simulink model "irep_force_control_simu_v2"  (R2015a)
settings: Solver=ode3  StartTime=0.0  StopTime=inf  FixedStep=dt  RelTol=1e-3
InitFcn:
  | IREP_DEPENDENCY
  | init_omni
  | init_filters
  | init_invivo
  | init_telemanipulation
  | init_parker_xyz
  | init_magnetic_tracker
  | init_loadcell
  | init_scopes
  | init_homing
  | init_force_control
  | init_xpc_invivo_simu
undefined symbols (not defined in the file or in its folder): ang_vel_scale, B_simu, beta, camera_home_voltage, counter_offset, dt, dt_trakstar, E_Y, encoder_counts, epsilon_robust_inverse, FS_LUT, gear_ratio, HomingFineEps, HomingRoughEps, HomingRoughVelocity, I1_primary, I1_secondary, I2_primary, I2_secondary, irep_parameters_left, irep_parameters_right, joystick_filter_coeffs, K_d, K_i, K_naive_inv, K_p, k_right, L1l, L1r, L2l, L2r, L_zeus, left_arm_home_voltage, left_x0_parallelogram, LeftArmHomingDirectionVector, LeftArmHomingIntGain, lin_vel_scale, LOADCELL_BIAS, LOADCELL_GAIN, max_conf_space_speed, N_joystick, N_pots, N_trakstar, OmegaMax, OmegaMin, orientation_epsilon, position_epsilon, pots_filter_coeffs, q_eps_backlash, quadrature_mode, r, right_arm_home_voltage, RightArmHomingDirectionVector, RightArmHomingIntGain, screw_pitch, statics_param, tau_compression_bias, tau_compression_gains, tau_neutral_deadband, tau_tension_bias ... (+15)
libraries: slrtlib x39, xpcrtudplib x13, xpcobsoletelib x13, simulink x8, dspswit3 x2, dspsigops x1
(part 3 of 6)

== system irep_force_control_simu_v2/In-Vivo System/motor simulation/q_des to q_cur mapping ==
  q cur in : Inport
  Bus Creator1 : BusCreator  Inputs=23
  Bus Selector : BusSelector  OutputSignals=Right arm - Proximal Segment Y,Right arm - Gripper Joint,Right arm - Proximal Segment X,Right arm - Distal Segment X,Right arm - Wrist Joint,Right arm - Distal Segment Y,Right arm - Parallelogram Deploy,Right arm - Parallelogram Insert,Left arm - Proximal Segment Y,Left arm - Gripper Joint,Left arm - Proximal Segment X,Left arm - Distal Segment X,Left arm - Wrist Joint,Left arm - Distal Segment Y,Left arm - Parallelogram Deploy,Left arm - Parallelogram Insert,Righ arm - Overall Translational Movement,Left arm - Overall Translational Movement,Camera shell open,Camera Pan,Camera Tilt,Parker insertion stage,Parker rotary stage
  Demux : Demux  Outputs=23
  Mux : Mux  Inputs=23
  q cur out : Outport
  wires:
  Demux/1 -> Bus Creator1/1  "Righ arm - Overall Translational Movement"
  Demux/2 -> Bus Creator1/2  "Right arm - Parallelogram Insert"
  Demux/3 -> Bus Creator1/3  "Right arm - Parallelogram Deploy"
  Demux/4 -> Bus Creator1/4  "Right arm - Proximal Segment X"
  Demux/5 -> Bus Creator1/5  "Right arm - Proximal Segment Y"
  Demux/6 -> Bus Creator1/6  "Right arm - Distal Segment X"
  Demux/7 -> Bus Creator1/7  "Right arm - Distal Segment Y"
  Demux/8 -> Bus Creator1/8  "Right arm - Wrist Joint"
  Demux/9 -> Bus Creator1/9  "Right arm - Gripper Joint"
  Demux/10 -> Bus Creator1/10  "Left arm - Overall Translational Movement"
  Demux/11 -> Bus Creator1/11  "Left arm - Parallelogram Insert"
  Demux/12 -> Bus Creator1/12  "Left arm - Parallelogram Deploy"
  Demux/13 -> Bus Creator1/13  "Left arm - Proximal Segment X"
  Demux/14 -> Bus Creator1/14  "Left arm - Proximal Segment Y"
  Demux/15 -> Bus Creator1/15  "Left arm - Distal Segment X"
  Demux/16 -> Bus Creator1/16  "Left arm - Distal Segment Y"
  Demux/17 -> Bus Creator1/17  "Left arm - Wrist Joint"
  Demux/18 -> Bus Creator1/18  "Left arm - Gripper Joint"
  Demux/19 -> Bus Creator1/19  "Camera shell open"
  Demux/20 -> Bus Creator1/20  "Camera Pan"
  Demux/21 -> Bus Creator1/21  "Camera Tilt"
  Demux/22 -> Bus Creator1/22  "Parker insertion stage"
  Demux/23 -> Bus Creator1/23  "Parker rotary stage"
  Bus Creator1/1 -> Bus Selector/1
  Bus Selector/1 -> Mux/1  "<Right arm - Proximal Segment Y>"
  Bus Selector/2 -> Mux/2  "<Right arm - Gripper Joint>"
  Bus Selector/3 -> Mux/3  "<Right arm - Proximal Segment X>"
  Bus Selector/4 -> Mux/4  "<Right arm - Distal Segment X>"
  Bus Selector/5 -> Mux/5  "<Right arm - Wrist Joint>"
  Bus Selector/6 -> Mux/6  "<Right arm - Distal Segment Y>"
  Bus Selector/7 -> Mux/7  "<Right arm - Parallelogram Deploy>"
  Bus Selector/8 -> Mux/8  "<Right arm - Parallelogram Insert>"
  Bus Selector/9 -> Mux/9  "<Left arm - Proximal Segment Y>"
  Bus Selector/10 -> Mux/10  "<Left arm - Gripper Joint>"
  Bus Selector/11 -> Mux/11  "<Left arm - Proximal Segment X>"
  Bus Selector/12 -> Mux/12  "<Left arm - Distal Segment X>"
  Bus Selector/13 -> Mux/13  "<Left arm - Wrist Joint>"
  Bus Selector/14 -> Mux/14  "<Left arm - Distal Segment Y>"
  Bus Selector/15 -> Mux/15  "<Left arm - Parallelogram Deploy>"
  Bus Selector/16 -> Mux/16  "<Left arm - Parallelogram Insert>"
  Bus Selector/17 -> Mux/17  "<Righ arm - Overall Translational Movement>"
  Bus Selector/18 -> Mux/18  "<Left arm - Overall Translational Movement>"
  Bus Selector/19 -> Mux/19  "<Camera shell open>"
  Bus Selector/20 -> Mux/20  "<Camera Pan>"
  Bus Selector/21 -> Mux/21  "<Camera Tilt>"
  Bus Selector/22 -> Mux/22  "<Parker insertion stage>"
  Bus Selector/23 -> Mux/23  "<Parker rotary stage>"
  q cur in/1 -> Demux/1
  Mux/1 -> q cur out/1

== system irep_force_control_simu_v2/In-Vivo System/motor simulation/u mapping ==
  u in : Inport
  Bus Selector : BusSelector  OutputSignals=Righ arm - Overall Translational Movement,Right arm - Parallelogram Insert,Right arm - Parallelogram Deploy,Right arm - Proximal Segment X,Right arm - Proximal Segment Y,Right arm - Distal Segment X,Right arm - Distal Segment Y,Right arm - Wrist Joint,Right arm - Gripper Joint,Left arm - Overall Translational Movement,Left arm - Parallelogram Insert,Left arm - Parallelogram Deploy,Left arm - Proximal Segment X,Left arm - Proximal Segment Y,Left arm - Distal Segment X,Left arm - Distal Segment Y,Left arm - Wrist Joint,Left arm - Gripper Joint,Camera shell open,Camera Pan,Camera Tilt,Parker insertion stage,Parker rotary stage
  Mux : Mux  Inputs=23
  u out : Outport
  wires:
  Bus Selector/1 -> Mux/1  "<Righ arm - Overall Translational Movement>"
  Bus Selector/2 -> Mux/2  "<Right arm - Parallelogram Insert>"
  Bus Selector/3 -> Mux/3  "<Right arm - Parallelogram Deploy>"
  Bus Selector/4 -> Mux/4  "<Right arm - Proximal Segment X>"
  Bus Selector/5 -> Mux/5  "<Right arm - Proximal Segment Y>"
  Bus Selector/6 -> Mux/6  "<Right arm - Distal Segment X>"
  Bus Selector/7 -> Mux/7  "<Right arm - Distal Segment Y>"
  Bus Selector/8 -> Mux/8  "<Right arm - Wrist Joint>"
  Bus Selector/9 -> Mux/9  "<Right arm - Gripper Joint>"
  Bus Selector/10 -> Mux/10  "<Left arm - Overall Translational Movement>"
  Bus Selector/11 -> Mux/11  "<Left arm - Parallelogram Insert>"
  Bus Selector/12 -> Mux/12  "<Left arm - Parallelogram Deploy>"
  Bus Selector/13 -> Mux/13  "<Left arm - Proximal Segment X>"
  Bus Selector/14 -> Mux/14  "<Left arm - Proximal Segment Y>"
  Bus Selector/15 -> Mux/15  "<Left arm - Distal Segment X>"
  Bus Selector/16 -> Mux/16  "<Left arm - Distal Segment Y>"
  Bus Selector/17 -> Mux/17  "<Left arm - Wrist Joint>"
  Bus Selector/18 -> Mux/18  "<Left arm - Gripper Joint>"
  Bus Selector/19 -> Mux/19  "<Camera shell open>"
  Bus Selector/20 -> Mux/20  "<Camera Pan>"
  Bus Selector/21 -> Mux/21  "<Camera Tilt>"
  Bus Selector/22 -> Mux/22  "<Parker insertion stage>"
  Bus Selector/23 -> Mux/23  "<Parker rotary stage>"
  u in/1 -> Bus Selector/1
  Mux/1 -> u out/1

== system irep_force_control_simu_v2/Joint Level PID Control in mm/Bus selector/Camera selector ==
  In1 : Inport
  Bus Selector : BusSelector  OutputSignals=q.Camera shell open,q.Camera Pan,q.Camera Tilt
  Mux : Mux  Inputs=3
  Out1 : Outport
  wires:
  Mux/1 -> Out1/1
  In1/1 -> Bus Selector/1
  Bus Selector/3 -> Mux/3  "<Camera Tilt>"
  Bus Selector/2 -> Mux/2  "<Camera Pan>"
  Bus Selector/1 -> Mux/1  "<Camera shell open>"

== system irep_force_control_simu_v2/Joint Level PID Control in mm/Bus selector/Left arm selector ==
  In1 : Inport
  Bus Selector : BusSelector  OutputSignals=q.Left arm - overall translational movement,q.Left arm - parallelogram insert joint,q.Left arm - parallelogram deployment joint,q.Left arm - proximal segment - bending in X,q.Left arm - proximal segment - bending in Y,q.Left arm - distal segment - bending in x,q.Left arm - distal segment - bending in y,q.Left arm - wrist,q.Left arm - gripper joint
  Mux : Mux  Inputs=9
  Out1 : Outport
  wires:
  In1/1 -> Bus Selector/1
  Mux/1 -> Out1/1
  Bus Selector/1 -> Mux/1  "<Left arm - overall translational movement>"
  Bus Selector/2 -> Mux/2  "<Left arm - parallelogram insert joint>"
  Bus Selector/3 -> Mux/3  "<Left arm - parallelogram deployment joint>"
  Bus Selector/4 -> Mux/4  "<Left arm - proximal segment - bending in X>"
  Bus Selector/5 -> Mux/5  "<Left arm - proximal segment - bending in Y>"
  Bus Selector/8 -> Mux/8  "<Left arm - wrist>"
  Bus Selector/9 -> Mux/9  "<Left arm - gripper joint>"
  Bus Selector/6 -> Mux/6  "<Left arm - distal segment - bending in x>"
  Bus Selector/7 -> Mux/7  "<Left arm - distal segment - bending in y>"

== system irep_force_control_simu_v2/Joint Level PID Control in mm/Bus selector/RZ ==
  In1 : Inport
  Bus Selector : BusSelector  OutputSignals=q.Parker insertion stage,q.Parker rotary stage
  Mux : Mux  Inputs=2
  Out1 : Outport
  wires:
  Mux/1 -> Out1/1
  In1/1 -> Bus Selector/1
  Bus Selector/2 -> Mux/2  "<Parker rotary stage>"
  Bus Selector/1 -> Mux/1  "<Parker insertion stage>"

== system irep_force_control_simu_v2/Joint Level PID Control in mm/Bus selector/Right arm selector ==
  In1 : Inport
  Bus Selector : BusSelector  OutputSignals=q.Right arm - overall translational movement,q.Right arm - parallelogram insert joint,q.Right arm - parallelogram deployment joint,q.Right arm - Proximal segment - bending in X,q.Righ arm - Proximal segment - bending in Y,q.Right arm - distal segment - bending in X,q.Right arm - distal segment - bending in Y,q.Right arm - wrist,q.Right arm - Gripper Joint
  Mux : Mux  Inputs=9
  Out1 : Outport
  wires:
  In1/1 -> Bus Selector/1
  Mux/1 -> Out1/1
  Bus Selector/1 -> Mux/1  "<Right arm - overall translational movement>"
  Bus Selector/2 -> Mux/2  "<Right arm - parallelogram insert joint>"
  Bus Selector/3 -> Mux/3  "<Right arm - parallelogram deployment joint>"
  Bus Selector/4 -> Mux/4  "<Right arm - Proximal segment - bending in X>"
  Bus Selector/5 -> Mux/5  "<Righ arm - Proximal segment - bending in Y>"
  Bus Selector/6 -> Mux/6  "<Right arm - distal segment - bending in X>"
  Bus Selector/7 -> Mux/7  "<Right arm - distal segment - bending in Y>"
  Bus Selector/8 -> Mux/8  "<Right arm - wrist>"
  Bus Selector/9 -> Mux/9  "<Right arm - Gripper Joint>"

== system irep_force_control_simu_v2/Scopes/Friction Estimation Data UDP/Right arm joint def ==
  sensors : Inport
  Bus Selector4 : BusSelector  OutputSignals=q.Right arm - overall translational movement,q.Right arm - parallelogram insert joint,q.Right arm - parallelogram deployment joint,q.Right arm - Proximal segment - bending in X,q.Righ arm - Proximal segment - bending in Y,q.Right arm - distal segment - bending in X,q.Right arm - distal segment - bending in Y,q.Right arm - wrist,q.Right arm - Gripper Joint
  Mux1 : Mux  Inputs=9
  right q_cur : Outport
  wires:
  Bus Selector4/1 -> Mux1/1  "<Right arm - overall translational movement>"
  Bus Selector4/2 -> Mux1/2  "<Right arm - parallelogram insert joint>"
  Bus Selector4/3 -> Mux1/3  "<Right arm - parallelogram deployment joint>"
  Bus Selector4/4 -> Mux1/4  "<Right arm - Proximal segment - bending in X>"
  Bus Selector4/5 -> Mux1/5  "<Righ arm - Proximal segment - bending in Y>"
  Bus Selector4/6 -> Mux1/6  "<Right arm - distal segment - bending in X>"
  Bus Selector4/7 -> Mux1/7  "<Right arm - distal segment - bending in Y>"
  Bus Selector4/8 -> Mux1/8  "<Right arm - wrist>"
  Bus Selector4/9 -> Mux1/9  "<Right arm - Gripper Joint>"
  sensors/1 -> Bus Selector4/1
  Mux1/1 -> right q_cur/1

== system irep_force_control_simu_v2/Trajectory Planner/Camera/Homing Procedure ==
  sensors : Inport
  Enable : EnablePort
  Bus Selector : BusSelector  OutputSignals=A/D signals.camera pots
  Discrete-Time Integrator : DiscreteIntegrator  InitialCondition=zeros(3,1)  SampleTime=dt
  Gain : Gain  Gain=[0.1 0.1 0.1]  SampleTime=dt
  Homing Completion : MATLAB Function  TreatAsAtomicUnit=on
  Sum : Sum  Inputs=|+-  SampleTime=dt
  Terminator1 : Terminator
  home voltage : Constant  Value=camera_home_voltage  SampleTime=dt
  q des : Outport
  wires:
  sensors/1 -> Bus Selector/1
  home voltage/1 -> Sum/1
  Bus Selector/1 -> Sum/2  "<camera pots>"
  Sum/1 -> Gain/1, Homing Completion/1(u)
  Gain/1 -> Discrete-Time Integrator/1
  Discrete-Time Integrator/1 -> q des/1
  Homing Completion/1(y) -> Terminator1/1

== system irep_force_control_simu_v2/Trajectory Planner/Camera/Joint Space ==
  Enable : EnablePort
  q des : Constant  Value=zeros(3,1)  SampleTime=dt
  Out1 : Outport
  wires:
  q des/1 -> Out1/1

== system irep_force_control_simu_v2/Trajectory Planner/Camera/Joystick Control for Cam ==
  sensors : Inport
  Enable : EnablePort
  Bus Selector : BusSelector  OutputSignals=A/D signals.camera joystick
  Demux : Demux  Outputs=3
  Discrete-Time Integrator : DiscreteIntegrator  SampleTime=dt  LimitOutput=on  UpperSaturationLimit=[3;3;3]  LowerSaturationLimit=[-3;-3;-3]
  Gain : Gain  Gain=diag([0.3 0.3 0.3])  Multiplication=Matrix(K*u)  SampleTime=dt
  Gain1 : Gain  Gain=-1
  Mux : Mux  Inputs=3
  q des : Outport
  wires:
  sensors/1 -> Bus Selector/1
  Gain/1 -> Discrete-Time Integrator/1
  Discrete-Time Integrator/1 -> q des/1
  Bus Selector/1 -> Demux/1  "<camera joystick>"
  Mux/1 -> Gain/1
  Demux/2 -> Gain1/1
  Demux/1 -> Mux/2
  Demux/3 -> Mux/1
  Gain1/1 -> Mux/3

== system irep_force_control_simu_v2/Trajectory Planner/Camera/Tool Tracking ==
  tool XY : Inport
  Enable : EnablePort
  Constant1 : Constant  Value=0  SampleTime=dt
  Discrete-Time Integrator : DiscreteIntegrator  SampleTime=dt  LimitOutput=on  UpperSaturationLimit=[3;3]  LowerSaturationLimit=[-3;-3]
  Gain : Gain  Gain=[0.01,0.01]  SampleTime=dt
  Mux : Mux  Inputs=2
  q des : Outport
  wires:
  tool XY/1 -> Gain/1
  Mux/1 -> q des/1
  Constant1/1 -> Mux/1
  Gain/1 -> Discrete-Time Integrator/1
  Discrete-Time Integrator/1 -> Mux/2

== system irep_force_control_simu_v2/Trajectory Planner/Left Arm/High Level ==
  Master : Inport
  sensors : Inport  Port=2
  Enable : EnablePort
  Actuation Compensation : Subsystem  TreatAsAtomicUnit=on
  Add : Sum
  Configuration Space : Subsystem  TreatAsAtomicUnit=on
  Enable Compensation : Constant  Value=0  SampleTime=dt
  Enable Configuration Space : Constant  Value=0  SampleTime=dt
  Enable Task Space : Constant  Value=0  SampleTime=dt
  Inverse Istantaneous Kinematics : Subsystem
  Merge : Merge  InitialOutput=zeros(8,1)
  Task Space : Subsystem  TreatAsAtomicUnit=on
  q des : Outport
  conf space : Outport  Port=2
  b0_dot_left : Outport  Port=3
  TASK_EN : Outport  Port=4
  current_pose : Outport  Port=5
  wires:
  Enable Task Space/1 -> TASK_EN/1, Task Space/Enable
  Task Space/1("b1 dot, psi dot") -> Merge/2
  Master/1 -> Task Space/1(Master), Inverse Istantaneous Kinematics/3(Master)
  Inverse Istantaneous Kinematics/2(conf space) -> Actuation Compensation/2(conf space), Task Space/2("b1 curr, psi curr"), conf space/1
  Inverse Istantaneous Kinematics/1(q des) -> Actuation Compensation/1(q des), Add/1
  Add/1 -> q des/1
  Actuation Compensation/1(epsilon) -> Add/2
  Enable Compensation/1 -> Actuation Compensation/Enable
  Enable Configuration Space/1 -> Configuration Space/Enable
  Configuration Space/1("b1 dot, psi dot") -> Merge/1
  sensors/1 -> Inverse Istantaneous Kinematics/2(sensors), Task Space/3(sensors)
  Merge/1 -> Inverse Istantaneous Kinematics/1(In1)
  Inverse Istantaneous Kinematics/3(b0 dot left) -> b0_dot_left/1
  Task Space/2(current_pose) -> current_pose/1

== system irep_force_control_simu_v2/Trajectory Planner/Left Arm/Low Level ==
  sensors : Inport
  Enable : EnablePort
  Bus Selector : BusSelector  OutputSignals=Pots_Connect.L_Pots_Connect
  Enable Home Procedure : Constant  Value=0  SampleTime=dt
  Enable Joint Space : Constant  Value=0  SampleTime=dt
  Home Procedure : Subsystem  TreatAsAtomicUnit=on
  Joint Space : Subsystem  TreatAsAtomicUnit=on
  Merge1 : Merge  InitialOutput=zeros(9,1)
  Not And : MATLAB Function  TreatAsAtomicUnit=on
  q des : Outport
  wires:
  sensors/1 -> Bus Selector/1, Home Procedure/1(sensors)
  Merge1/1 -> q des/1
  Enable Joint Space/1 -> Joint Space/Enable
  Joint Space/1(q des) -> Merge1/2
  Bus Selector/1 -> Not And/1(connected)  "<L_Pots_Connect>"
  Enable Home Procedure/1 -> Not And/2(enable_home)
  Not And/1(enable) -> Home Procedure/Enable
  Home Procedure/1(q des) -> Merge1/1

== system irep_force_control_simu_v2/Trajectory Planner/RZ/Joystick Control for RZ ==
  sensors : Inport
  Enable : EnablePort
  Bus Selector : BusSelector  OutputSignals=A/D signals.camera joystick
  Embedded MATLAB Function : MATLAB Function  TreatAsAtomicUnit=on
  Gain : Gain  Gain=diag(-[2 0 0.005])  Multiplication=Matrix(K*u)  SampleTime=dt
  q des : Outport
  wires:
  sensors/1 -> Bus Selector/1
  Gain/1 -> q des/1
  Embedded MATLAB Function/1(y) -> Gain/1
  Bus Selector/1 -> Embedded MATLAB Function/1(u)  "<camera joystick>"

== system irep_force_control_simu_v2/Trajectory Planner/RZ/Subsystem ==
  In1 : Inport
  Demux : Demux  Outputs=3
  Mux : Mux  Inputs=2
  Terminator : Terminator
  Out1 : Outport
  wires:
  Demux/1 -> Mux/1
  Demux/3 -> Mux/2
  Demux/2 -> Terminator/1
  In1/1 -> Demux/1
  Mux/1 -> Out1/1

== system irep_force_control_simu_v2/Trajectory Planner/Right Arm/High Level ==
  Master : Inport
  sensors : Inport  Port=2
  Enable : EnablePort
  Actuation Compensation : Subsystem  TreatAsAtomicUnit=on
  Add : Sum
  Configuration Space : Subsystem  TreatAsAtomicUnit=on
  Enable Compensation : Constant  Value=0  SampleTime=dt
  Enable Configuration Space : Constant  Value=0  SampleTime=dt
  Enable Task Space : Constant  Value=0  SampleTime=dt
  Inverse Istantaneous Kinematics : Subsystem
  Merge : Merge  InitialOutput=zeros(8,1)
  Right eps : slrtlib/Displays and Logging/Scope   scopeno=32  scopetype=Host  autostart=on  viewmode=Numerical  formatstr=scope_format_right_q_des  grid=on  ylimits=[0,0]  nosamples=10  noprepostsamples=0  interleave=1  triggermode=FreeRun  triggersignal=1  trigsignalfromport=off  triggerlevel=0.0  triggerslope=Either  triggerscope=1  triggersample=0  filename=weights.dat  mode=Lazy  writesize=512  autorestart=off  dynamicfilemode=off  maxwritefilesize=512*1024^2
  Task Space : Subsystem  TreatAsAtomicUnit=on
  delay : Subsystem
  q des : Outport
  conf space : Outport  Port=2  PortDimensions=8
  b0 dot : Outport  Port=3  PortDimensions=1
  TASK_EN : Outport  Port=4
  current_pose : Outport  Port=5
  q dot sgn : Outport  Port=6
  wires:
  Merge/1 -> [psi_dot], Inverse Istantaneous Kinematics/1(PSI dot)
  Enable Task Space/1 -> TASK_EN/1, Task Space/Enable
  Task Space/1("b0 dot, b1 dot, psi dot") -> Merge/2
  Master/1 -> Task Space/1(Master), Inverse Istantaneous Kinematics/3(Master)
  Inverse Istantaneous Kinematics/2(conf space) -> Actuation Compensation/2(conf space), Task Space/2("b1 curr, psi curr"), conf space/1
  Configuration Space/1("b1 dot, psi dot") -> Merge/1
  Inverse Istantaneous Kinematics/1(q des) -> Add/1, delay/1(In1)
  Actuation Compensation/1(epsilon) -> Add/2, Right eps/1
  Enable Compensation/1 -> Actuation Compensation/Enable
  sensors/1 -> Task Space/3(sensors), Inverse Istantaneous Kinematics/2(sensors)
  Inverse Istantaneous Kinematics/3(b0_dot_right) -> b0 dot/1
  Add/1 -> q des/1
  Task Space/2(current_pose) -> current_pose/1
  Enable Configuration Space/1 -> Configuration Space/Enable
  [psi_dot] -> Actuation Compensation/3(psi dot)
  delay/1(Out1) -> Actuation Compensation/1(q des)
  Actuation Compensation/2(q dot sgn) -> q dot sgn/1

== system irep_force_control_simu_v2/Trajectory Planner/Right Arm/Low Level ==
  sensors : Inport
  Enable : EnablePort
  Bus Selector : BusSelector  OutputSignals=Pots_Connect.R_Pots_Connect
  Enable Home Procedure : Constant  Value=0  SampleTime=dt
  Enable Joint Space : Constant  Value=0  SampleTime=dt
  Home Procedure : Subsystem  TreatAsAtomicUnit=on
  Joint Space : Subsystem  TreatAsAtomicUnit=on
  Merge1 : Merge  InitialOutput=zeros(9,1)
  Not And : MATLAB Function  TreatAsAtomicUnit=on
  q des : Outport
  wires:
  sensors/1 -> Home Procedure/1(sensors), Bus Selector/1
  Home Procedure/1(q des) -> Merge1/1
  Enable Joint Space/1 -> Joint Space/Enable
  Joint Space/1(q des) -> Merge1/2
  Merge1/1 -> q des/1
  Bus Selector/1 -> Not And/1(connected)  "<R_Pots_Connect>"
  Not And/1(enable) -> Home Procedure/Enable
  Enable Home Procedure/1 -> Not And/2(enable_home)

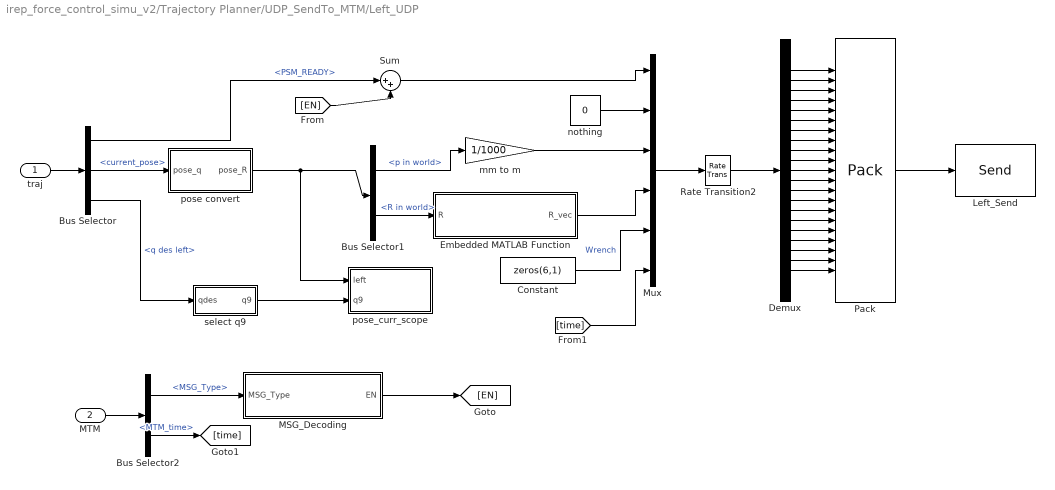
== system irep_force_control_simu_v2/Trajectory Planner/UDP_SendTo_MTM/Left_UDP ==
  traj : Inport
  MTM : Inport  Port=2
  Bus Selector : BusSelector  OutputSignals=left arm.PSM_READY,left arm.current_pose,left arm.q des left
  Bus Selector1 : BusSelector  OutputSignals=p in world,R in world
  Bus Selector2 : BusSelector  OutputSignals=MSG_Type,MTM_time
  Constant : Constant  Value=zeros(6,1)
  Demux : Demux  Outputs=21
  Embedded MATLAB Function : MATLAB Function  TreatAsAtomicUnit=on
  Left_Send : xpcrtudplib/Legacy UDP/Send   ipAddress=192.168.1.104  ipPort=10004  localPort=-1  vblLen=off  sampletime=dt_omni
  MSG_Decoding : MATLAB Function  TreatAsAtomicUnit=on
  Mux : Mux  Inputs=6
  Pack : xpcobsoletelib/Utilities/Pack   datatypes={'double' 'double' 'double' 'double' 'double' 'double' 'double' 'double' 'double' 'double' 'double' 'double' 'double' 'double' 'double' 'double' 'double' 'double' 'double' 'double' 'double'}  byteAlign=1
  Rate Transition2 : RateTransition  OutPortSampleTime=dt_omni
  Sum : Sum  Inputs=|++
  mm to m : Gain  Gain=1/1000
  nothing : Constant  Value=0
  pose convert : Subsystem
  pose_curr_scope : Subsystem
  select q9 : Subsystem
  wires:
  pose convert/1(pose_R) -> Bus Selector1/1, pose_curr_scope/1(left)
  Bus Selector/2 -> pose convert/1(pose_q)  "<current_pose>"
  Constant/1 -> Mux/5  "Wrench"
  Demux/21 -> Pack/21
  Demux/20 -> Pack/20
  Demux/19 -> Pack/19
  Demux/18 -> Pack/18
  Demux/17 -> Pack/17
  Demux/16 -> Pack/16
  Demux/15 -> Pack/15
  Demux/14 -> Pack/14
  Demux/13 -> Pack/13
  Demux/12 -> Pack/12
  Demux/11 -> Pack/11
  Demux/10 -> Pack/10
  Demux/9 -> Pack/9
  Demux/8 -> Pack/8
  Demux/7 -> Pack/7
  Demux/6 -> Pack/6
  Demux/5 -> Pack/5
  Demux/4 -> Pack/4
  Demux/3 -> Pack/3
  Demux/2 -> Pack/2
  Demux/1 -> Pack/1
  [time] -> Mux/6
  Sum/1 -> Mux/1
  [EN] -> Sum/2
  Bus Selector/1 -> Sum/1  "<PSM_READY>"
  nothing/1 -> Mux/2
  MSG_Decoding/1(EN) -> [EN]
  Bus Selector2/2 -> [time]  "<MTM_time>"
  Bus Selector2/1 -> MSG_Decoding/1(MSG_Type)  "<MSG_Type>"
  MTM/1 -> Bus Selector2/1
  select q9/1(q9) -> pose_curr_scope/2(q9)
  Bus Selector/3 -> select q9/1(qdes)  "<q des left>"
  mm to m/1 -> Mux/3
  traj/1 -> Bus Selector/1
  Embedded MATLAB Function/1(R_vec) -> Mux/4
  Bus Selector1/1 -> mm to m/1  "<p in world>"
  Rate Transition2/1 -> Demux/1
  Mux/1 -> Rate Transition2/1
  Pack/1 -> Left_Send/1
  Bus Selector1/2 -> Embedded MATLAB Function/1(R)  "<R in world>"

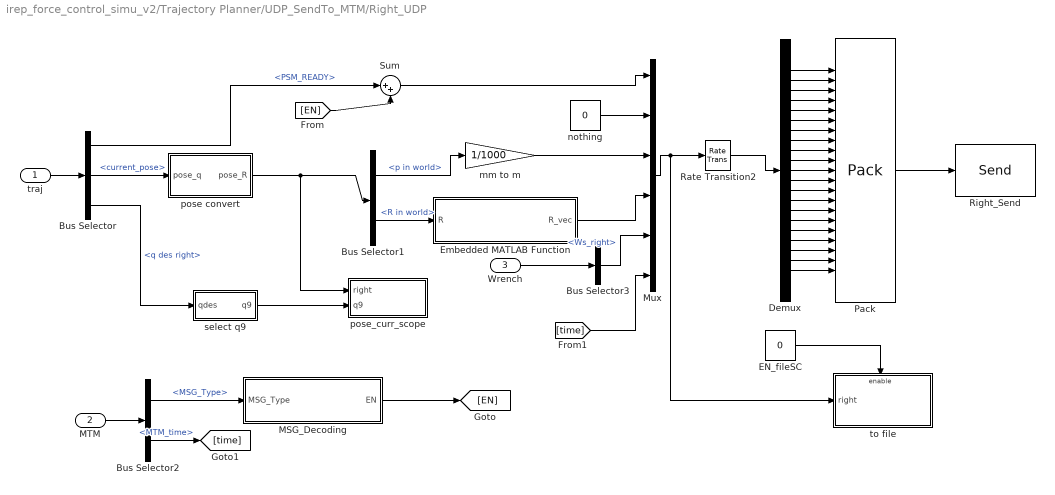
== system irep_force_control_simu_v2/Trajectory Planner/UDP_SendTo_MTM/Right_UDP ==
  traj : Inport
  MTM : Inport  Port=2
  Wrench : Inport  Port=3
  Bus Selector : BusSelector  OutputSignals=right arm.PSM_READY,right arm.current_pose,right arm.q des right
  Bus Selector1 : BusSelector  OutputSignals=p in world,R in world
  Bus Selector2 : BusSelector  OutputSignals=MSG_Type,MTM_time
  Bus Selector3 : BusSelector  OutputSignals=Ws_right
  Demux : Demux  Outputs=21
  EN_fileSC : Constant  Value=0
  Embedded MATLAB Function : MATLAB Function  TreatAsAtomicUnit=on
  MSG_Decoding : MATLAB Function  TreatAsAtomicUnit=on
  Mux : Mux  Inputs=6
  Pack : xpcobsoletelib/Utilities/Pack   datatypes={'double' 'double' 'double' 'double' 'double' 'double' 'double' 'double' 'double' 'double' 'double' 'double' 'double' 'double' 'double' 'double' 'double' 'double' 'double' 'double' 'double'}  byteAlign=1
  Rate Transition2 : RateTransition  OutPortSampleTime=dt_omni
  Right_Send : xpcrtudplib/Legacy UDP/Send   ipAddress=192.168.1.104  ipPort=10005  localPort=-1  vblLen=off  sampletime=dt_omni
  Sum : Sum  Inputs=|++
  mm to m : Gain  Gain=1/1000
  nothing : Constant  Value=0
  pose convert : Subsystem
  pose_curr_scope : Subsystem
  select q9 : Subsystem
  to file : Subsystem
  wires:
  Bus Selector1/2 -> Embedded MATLAB Function/1(R)  "<R in world>"
  Pack/1 -> Right_Send/1
  Mux/1 -> Rate Transition2/1, to file/1(right)
  Rate Transition2/1 -> Demux/1
  Bus Selector1/1 -> mm to m/1  "<p in world>"
  Embedded MATLAB Function/1(R_vec) -> Mux/4
  traj/1 -> Bus Selector/1
  mm to m/1 -> Mux/3
  Bus Selector/3 -> select q9/1(qdes)  "<q des right>"
  select q9/1(q9) -> pose_curr_scope/2(q9)
  MTM/1 -> Bus Selector2/1
  Bus Selector2/1 -> MSG_Decoding/1(MSG_Type)  "<MSG_Type>"
  Bus Selector2/2 -> [time]  "<MTM_time>"
  MSG_Decoding/1(EN) -> [EN]
  EN_fileSC/1 -> to file/Enable
  nothing/1 -> Mux/2
  Bus Selector/1 -> Sum/1  "<PSM_READY>"
  [EN] -> Sum/2
  Sum/1 -> Mux/1
  [time] -> Mux/6
  Demux/1 -> Pack/1
  Demux/2 -> Pack/2
  Demux/3 -> Pack/3
  Demux/4 -> Pack/4
  Demux/5 -> Pack/5
  Demux/6 -> Pack/6
  Demux/7 -> Pack/7
  Demux/8 -> Pack/8
  Demux/9 -> Pack/9
  Demux/10 -> Pack/10
  Demux/11 -> Pack/11
  Demux/12 -> Pack/12
  Demux/13 -> Pack/13
  Demux/14 -> Pack/14
  Demux/15 -> Pack/15
  Demux/16 -> Pack/16
  Demux/17 -> Pack/17
  Demux/18 -> Pack/18
  Demux/19 -> Pack/19
  Demux/20 -> Pack/20
  Demux/21 -> Pack/21
  Wrench/1 -> Bus Selector3/1
  Bus Selector3/1 -> Mux/5  "<Ws_right>"
  Bus Selector/2 -> pose convert/1(pose_q)  "<current_pose>"
  pose convert/1(pose_R) -> Bus Selector1/1, pose_curr_scope/1(right)

== system irep_force_control_simu_v2/Wrench Estimation/Wrench Est Right Arm/sel param ==
  note: irep_parameters_right = [Y_OFFSET;L1r;L2r;p_gripper];
  In : Inport
  Demux : Demux  Outputs=[1,1,1,3]
  Mux1 : Mux  Inputs=2
  Terminator : Terminator
  Terminator1 : Terminator
  L : Outport
  wires:
  In/1 -> Demux/1
  Mux1/1 -> L/1
  Demux/2 -> Mux1/1  "L1"
  Demux/3 -> Mux1/2  "L2"
  Demux/1 -> Terminator/1  "Y_OFFSET"
  Demux/4 -> Terminator1/1  "p_gripper"

== system irep_force_control_simu_v2/Wrench Estimation/tau sensing compensation/tau sensing compensation LUT ==
  note: 1st Segment tau bias
  note: 2nd Segment tau bias
  note: Inputs
  tau_measured : Inport
  q_dot_sign : Inport  Port=2
  psi : Inport  Port=3
  Enable : EnablePort
  Constant : Constant  Value=zeros(4,1)
  Demux : Demux  Outputs=[4,4]
  Demux1 : Demux  Outputs=[2,2]
  Mux : Mux  Inputs=2
  Sum : Sum  Inputs=|+-
  Terminator : Terminator
  Terminator1 : Terminator
  tau seg2 bias LUT : Subsystem
  tau_comp : Outport
  wires:
  psi/1 -> Demux1/1
  q_dot_sign/1 -> Demux/1
  Demux1/1 -> [psi1]
  Demux1/2 -> [psi2]
  [psi1] -> Terminator/1
  Demux/1 -> [qdot_sgn1]
  Demux/2 -> [qdot_sgn2]
  [qdot_sgn1] -> Terminator1/1
  tau_measured/1 -> [tau_measured]
  [psi2] -> tau seg2 bias LUT/2(psi seg2)
  [qdot_sgn2] -> tau seg2 bias LUT/1(q dot seg2)
  Constant/1 -> Mux/1
  tau seg2 bias LUT/1(tau bias seg2) -> Mux/2
  Mux/1 -> Sum/2  "tau bias"
  [tau_measured] -> Sum/1
  Sum/1 -> tau_comp/1

== system irep_force_control_simu_v2/Wrench Estimation/tau sensing compensation/tau sensing compensation gain model ==
  q_bb : Inport
  tau_sensed : Inport  Port=2
  Enable : EnablePort
  friction compensation : MATLAB Function  TreatAsAtomicUnit=on
  tau_compression_bias : Constant  Value=tau_compression_bias
  tau_compression_gains : Constant  Value=tau_compression_gains
  tau_neutral_deadband : Constant  Value=tau_neutral_deadband
  tau_tension_bias : Constant  Value=tau_tension_bias
  tau_tension_gains : Constant  Value=tau_tension_gains
  tau_comp : Outport
  wires:
  tau_neutral_deadband/1 -> friction compensation/7(deadband)
  tau_compression_gains/1 -> friction compensation/4(gain_compression)
  tau_tension_gains/1 -> friction compensation/3(gain_tension)
  tau_sensed/1 -> friction compensation/2(tau_sensed)
  q_bb/1 -> friction compensation/1(q_bb)
  friction compensation/1(tau_comp) -> tau_comp/1
  tau_tension_bias/1 -> friction compensation/5(bias_tension)
  tau_compression_bias/1 -> friction compensation/6(bias_compression)

== system irep_force_control_simu_v2/In-Vivo System/Magnetic Tracker 125 Hz/process trak1/Filter1 ==
  in : Inport
  Discrete FIR Filter : DiscreteFir  CoefSource=Input port  SampleTime=dt_trakstar  AccumDataTypeStr=Inherit: Same as product output
  Gain : Gain  Gain=1/N_trakstar  SampleTime=dt_trakstar
  trakstar_filter_coeffs : Constant  Value=trakstar_filter_coeffs  SampleTime=dt_trakstar
  out : Outport
  wires:
  Gain/1 -> out/1
  in/1 -> Discrete FIR Filter/1
  Discrete FIR Filter/1 -> Gain/1
  trakstar_filter_coeffs/1 -> Discrete FIR Filter/2

== system irep_force_control_simu_v2/In-Vivo System/Magnetic Tracker 125 Hz/process trak2/Filter1 ==
  in : Inport
  Discrete FIR Filter : DiscreteFir  CoefSource=Input port  SampleTime=dt_trakstar  AccumDataTypeStr=Inherit: Same as product output
  Gain : Gain  Gain=1/N_trakstar  SampleTime=dt_trakstar
  trakstar_filter_coeffs : Constant  Value=trakstar_filter_coeffs  SampleTime=dt_trakstar
  out : Outport
  wires:
  trakstar_filter_coeffs/1 -> Discrete FIR Filter/2
  Discrete FIR Filter/1 -> Gain/1
  in/1 -> Discrete FIR Filter/1
  Gain/1 -> out/1

== system irep_force_control_simu_v2/In-Vivo System/Magnetic Tracker 125 Hz/process trak3/Filter1 ==
  in : Inport
  Discrete FIR Filter : DiscreteFir  CoefSource=Input port  SampleTime=dt_trakstar  AccumDataTypeStr=Inherit: Same as product output
  Gain : Gain  Gain=1/N_trakstar  SampleTime=dt_trakstar
  trakstar_filter_coeffs : Constant  Value=trakstar_filter_coeffs  SampleTime=dt_trakstar
  out : Outport
  wires:
  Gain/1 -> out/1
  in/1 -> Discrete FIR Filter/1
  Discrete FIR Filter/1 -> Gain/1
  trakstar_filter_coeffs/1 -> Discrete FIR Filter/2

== system irep_force_control_simu_v2/In-Vivo System/Magnetic Tracker 125 Hz/process trak4/Filter1 ==
  in : Inport
  Discrete FIR Filter : DiscreteFir  CoefSource=Input port  SampleTime=dt_trakstar  AccumDataTypeStr=Inherit: Same as product output
  Gain : Gain  Gain=1/N_trakstar  SampleTime=dt_trakstar
  trakstar_filter_coeffs : Constant  Value=trakstar_filter_coeffs  SampleTime=dt_trakstar
  out : Outport
  wires:
  trakstar_filter_coeffs/1 -> Discrete FIR Filter/2
  Discrete FIR Filter/1 -> Gain/1
  in/1 -> Discrete FIR Filter/1
  Gain/1 -> out/1

== system irep_force_control_simu_v2/Trajectory Planner/Left Arm/High Level/Actuation Compensation ==
  q des : Inport
  conf space : Inport  Port=2
  Enable : EnablePort
  1/stiffness : Gain  Gain=K_naive_inv  Multiplication=Matrix(K*u)  SampleTime=dt
  Compute Taus : Subsystem
  Grad U1 : Subsystem
  Grad U2 : Subsystem
  Mux : Mux  Inputs=2
  Mux1 : Mux  Inputs=3
  Parallelogram Backlash Compensatior : Subsystem  TreatAsAtomicUnit=on
  comp perc : Gain  Gain=diag([0.8 0.8 0.8 0.8])  Multiplication=Matrix(K*u)  SampleTime=dt
  padding 2 for wrist and gripper : Constant  Value=zeros(2,1)  SampleTime=dt
  epsilon : Outport
  wires:
  conf space/1 -> Grad U1/1(conf space), Compute Taus/2(In2), Grad U2/1(conf space)
  q des/1 -> Grad U2/2(q), Grad U1/2(q), Parallelogram Backlash Compensatior/1(q des)
  Grad U1/1(grad_U) -> Mux/1
  Grad U2/1(grad_U) -> Mux/2
  Mux/1 -> Compute Taus/1(In1)
  Compute Taus/1(tau) -> 1/stiffness/1
  Parallelogram Backlash Compensatior/1(epsilon) -> Mux1/1
  1/stiffness/1 -> comp perc/1  "epsilon"
  padding 2 for wrist and gripper/1 -> Mux1/3
  comp perc/1 -> Mux1/2
  Mux1/1 -> epsilon/1

== system irep_force_control_simu_v2/Trajectory Planner/Left Arm/High Level/Configuration Space ==
  Enable : EnablePort
  Enable Parallelogram : Constant  Value=0  SampleTime=dt
  Enable Stem : Constant  Value=0  SampleTime=dt
  Mux : Mux  Inputs=3
  Parallelogram : Subsystem  TreatAsAtomicUnit=on
  Stem : Subsystem  TreatAsAtomicUnit=on
  b0 : Constant  Value=0  SampleTime=dt
  "b1 dot, psi dot" : Outport  InitialOutput=zeros(8,1)
  wires:
  Enable Stem/1 -> Stem/Enable
  Enable Parallelogram/1 -> Parallelogram/Enable
  Mux/1 -> "b1 dot, psi dot"/1
  b0/1 -> Mux/1
  Parallelogram/1(b1) -> Mux/2
  Stem/1(psi dot) -> Mux/3

== system irep_force_control_simu_v2/Trajectory Planner/Left Arm/High Level/Inverse Istantaneous Kinematics ==
  In1 : Inport
  sensors : Inport  Port=2
  Master : Inport  Port=3
  5-Bar Inverse Kinematics : MATLAB Function  TreatAsAtomicUnit=on
  Bus Creator : BusCreator  Inputs=3
  Bus Creator1 : BusCreator
  Bus Selector : BusSelector  OutputSignals=q.Parker insertion stage
  Coordination Module : Subsystem
  Demux : Demux  Outputs=[1 2 5]
  Enable Gripper : Constant  Value=0  SampleTime=dt
  Integrator 3 : DiscreteIntegrator  InitialCondition=[left_x0_parallelogram z0_parallelogram]  SampleTime=dt  LimitOutput=on  UpperSaturationLimit=[-x0_parallelogram z0_parallelogram_max]  LowerSaturationLimit=[-x0_parallelogram_max z0_parallelogram]
  Integrator 4 : DiscreteIntegrator  InitialCondition=[pi/2;0;pi/2;0;0]  SampleTime=dt  LimitOutput=on  UpperSaturationLimit=[theta_max inf theta_max inf wrist_max]  LowerSaturationLimit=[theta_min1 -inf theta_min2 -inf wrist_min]
  Jaw Open/Close Module : Subsystem  TreatAsAtomicUnit=on
  Saturation : Saturate  UpperLimit=20  LowerLimit=0
  Snake inverse kinematics : MATLAB Function  TreatAsAtomicUnit=on
  q des : Outport
  conf space : Outport  Port=2
  b0 dot left : Outport  Port=3
  wires:
  Integrator 4/1 -> Snake inverse kinematics/1(psi), Bus Creator/3  "psi curr"
  Bus Creator/1 -> conf space/1
  In1/1 -> Demux/1
  Bus Creator1/1 -> q des/1
  Jaw Open/Close Module/1(q9) -> Bus Creator1/4  "q9"
  Coordination Module/2("q2, q3") -> Bus Creator1/2  "q2, q3"
  Coordination Module/1(q1) -> Saturation/1  "q1"
  Integrator 3/1 -> 5-Bar Inverse Kinematics/1(b1), Coordination Module/1(b1), Bus Creator/2  "b1 curr"
  5-Bar Inverse Kinematics/1(q) -> Coordination Module/2(q par)
  sensors/1 -> Bus Selector/1
  Enable Gripper/1 -> Jaw Open/Close Module/Enable
  Saturation/1 -> Bus Creator1/1
  Snake inverse kinematics/1(q) -> Bus Creator1/3
  Bus Selector/1 -> Bus Creator/1  "<Parker insertion stage>"
  Demux/3 -> Integrator 4/1
  Demux/2 -> Integrator 3/1  "psi dot"
  Demux/1 -> b0 dot left/1  "b1 dot"
  Master/1 -> Jaw Open/Close Module/1(sensors)

== system irep_force_control_simu_v2/Trajectory Planner/Left Arm/High Level/Task Space ==
  note: IREP Task Space Module v 0.2 - © 2011 Andrea Bajo, Nabil Simaan
  Master : Inport
  "b1 curr, psi curr" : Inport  Port=2
  sensors : Inport  Port=3
  Enable : EnablePort
  Bus Creator : BusCreator  Inputs=2
  Bus Selector : BusSelector  OutputSignals=p in world,R in world
  Compute Weigths : Subsystem  TreatAsAtomicUnit=on
  Desired Twist Module : Subsystem
  Direct Kinematics IREP : Subsystem  TreatAsAtomicUnit=on
  Jxpsi Inverse IREP : Subsystem  TreatAsAtomicUnit=on
  Receive Desired Pose from MTM : Subsystem
  pose cur quat : MATLAB Function  TreatAsAtomicUnit=on
  right task space scope : Subsystem
  "b1 dot, psi dot" : Outport  PortDimensions=8  InitialOutput=zeros(8,1)
  current_pose : Outport  Port=2  PortDimensions=7  InitialOutput=[zeros(3,1);1;0;0;0]
  wires:
  "b1 curr, psi curr"/1 -> Direct Kinematics IREP/1("b1, psi"), Jxpsi Inverse IREP/3("b1, psi"), Compute Weigths/2(conf space)
  Receive Desired Pose from MTM/1("pose, flags") -> Desired Twist Module/2(des pose), [L_pose_des]
  Direct Kinematics IREP/1(Current Pose) -> Desired Twist Module/1(current pose), Bus Selector/1
  Master/1 -> Receive Desired Pose from MTM/1(Master)
  Jxpsi Inverse IREP/1(conf dot des) -> "b1 dot, psi dot"/1
  Desired Twist Module/1(x des) -> Jxpsi Inverse IREP/1(x des)
  Compute Weigths/1(weights) -> Jxpsi Inverse IREP/2(weights)
  [L_pose_des] -> right task space scope/1(In)
  sensors/1 -> Compute Weigths/1(sensors)
  Bus Selector/1 -> Bus Creator/1  "<p in world>"
  Bus Selector/2 -> pose cur quat/1(R)  "<R in world>"
  pose cur quat/1(quat) -> Bus Creator/2
  Bus Creator/1 -> current_pose/1

== system irep_force_control_simu_v2/Trajectory Planner/Left Arm/Low Level/Home Procedure ==
  sensors : Inport
  Enable : EnablePort
  Bus Selector : BusSelector  OutputSignals=A/D signals.left arm pots
  Demux : Demux  Outputs=[9 1]
  Fine Homing - Integral Control : Subsystem
  Fine_Rough_Homing_Switch : MATLAB Function  TreatAsAtomicUnit=on
  Homing Direction : Gain  Gain=diag(LeftArmHomingDirectionVector)  Multiplication=Matrix(K*u)  SampleTime=dt
  Homing Flags : Subsystem
  HomingRoughEps : Constant  Value=HomingRoughEps  SampleTime=dt
  HomingRoughVelocity : Constant  Value=HomingRoughVelocity  SampleTime=dt
  Select Homing Joint : Gain  Gain=diag([1;1;1;1;1;1;1;1;1])  Multiplication=Matrix(K*u)  SampleTime=dt
  Sum : Sum  Inputs=|+-  SampleTime=dt
  Sum1 : Sum  Inputs=|++
  Terminator : Terminator
  Unit Delay : UnitDelay  InitialCondition=zeros(9,1)  SampleTime=-1
  Unit Delay1 : UnitDelay  InitialCondition=false(9,1)  SampleTime=-1
  dt : Constant  Value=dt  SampleTime=dt
  home voltage : Constant  Value=left_arm_home_voltage  SampleTime=dt
  q des : Outport  InitialOutput=zeros(9,1)
  wires:
  sensors/1 -> Bus Selector/1
  Sum/1 -> Select Homing Joint/1
  home voltage/1 -> Sum/1
  Bus Selector/1 -> Demux/1  "<left arm pots>"
  Demux/1 -> Sum/2
  Demux/2 -> Terminator/1
  Select Homing Joint/1 -> Homing Direction/1
  HomingRoughVelocity/1 -> Fine_Rough_Homing_Switch/4(HomingVel)
  Unit Delay1/1 -> Fine_Rough_Homing_Switch/6(PrevHomedJoint)
  Fine_Rough_Homing_Switch/3(HomedJoint) -> Unit Delay1/1
  HomingRoughEps/1 -> Fine_Rough_Homing_Switch/3(ERROR_eps)
  dt/1 -> Fine_Rough_Homing_Switch/2(dt)
  Unit Delay/1 -> Fine_Rough_Homing_Switch/5(q_cur)
  Fine_Rough_Homing_Switch/2(q_des) -> Unit Delay/1, Sum1/2
  Fine_Rough_Homing_Switch/1(EnableFineHoming) -> Fine Homing - Integral Control/Enable
  Fine Homing - Integral Control/1(q_des_fine) -> Sum1/1
  Sum1/1 -> q des/1
  Homing Direction/1 -> Fine_Rough_Homing_Switch/1(error), Fine Homing - Integral Control/1(error), Homing Flags/1(u)

== system irep_force_control_simu_v2/Trajectory Planner/Left Arm/Low Level/Joint Space ==
  Enable : EnablePort
  q desired : Constant  Value=zeros(9,1)  SampleTime=dt
  q des : Outport
  wires:
  q desired/1 -> q des/1

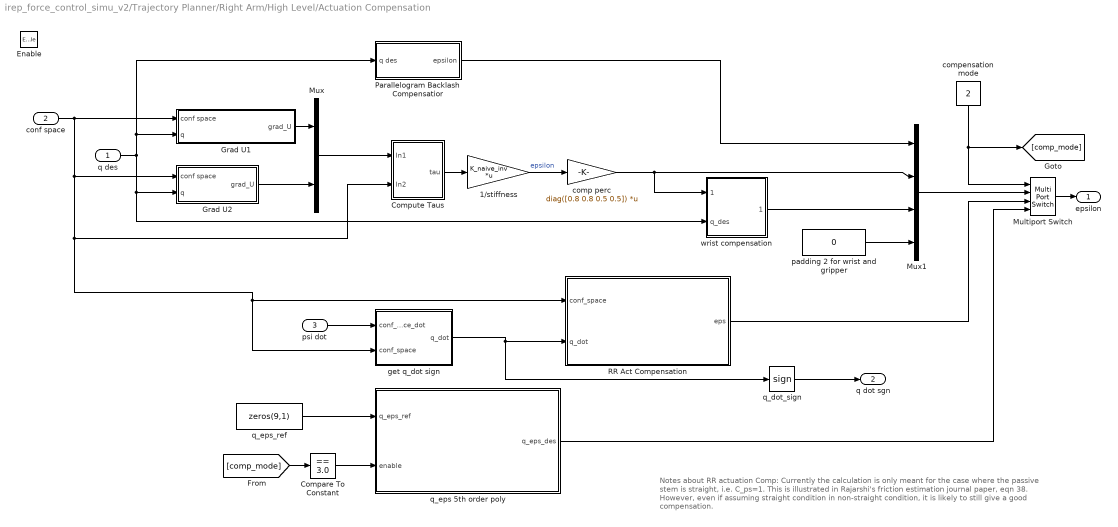
== system irep_force_control_simu_v2/Trajectory Planner/Right Arm/High Level/Actuation Compensation ==
  note: Notes about RR actuation Comp:
      | Currently the calculation is only meant for the case where the passive stem is straight, i.e. C_ps=1.
      | This is illustrated in Rajarshi's friction estimation journal paper, eqn 38.
      | However, even if assuming straight condition in non-straight condition,
      | it is likely to still give a good compensation.
  q des : Inport
  conf space : Inport  Port=2
  psi dot : Inport  Port=3
  Enable : EnablePort
  1/stiffness : Gain  Gain=K_naive_inv  Multiplication=Matrix(K*u)  SampleTime=dt
  Compare To Constant : simulink/Logic and Bit Operations/Compare To Constant  relop===  const=3.0  OutDataTypeStr=uint8
  Compute Taus : Subsystem
  Grad U1 : Subsystem
  Grad U2 : Subsystem
  Multiport Switch : MultiPortSwitch
  Mux : Mux  Inputs=2
  Mux1 : Mux
  Parallelogram Backlash Compensatior : Subsystem  TreatAsAtomicUnit=on
  RR Act Compensation : MATLAB Function  TreatAsAtomicUnit=on
  comp perc : Gain  Gain=diag([0.8 0.8 0.5 0.5])  Multiplication=Matrix(K*u)  SampleTime=dt
  compensation mode : Constant  Value=2
  get q_dot sign : Subsystem
  padding 2 for wrist and gripper : Constant  Value=0  SampleTime=dt
  q_dot_sign : Signum
  q_eps 5th order poly : Subsystem
  q_eps_ref : Constant  Value=zeros(9,1)  SampleTime=dt
  wrist compensation : MATLAB Function  TreatAsAtomicUnit=on
  epsilon : Outport
  q dot sgn : Outport  Port=2
  wires:
  conf space/1 -> Grad U1/1(conf space), Grad U2/1(conf space), Compute Taus/2(In2), RR Act Compensation/1(conf_space), get q_dot sign/2(conf_space)
  q des/1 -> Grad U1/2(q), Parallelogram Backlash Compensatior/1(q des), Grad U2/2(q), wrist compensation/2(q_des)
  Grad U1/1(grad_U) -> Mux/1
  Grad U2/1(grad_U) -> Mux/2
  Mux/1 -> Compute Taus/1(In1)
  Compute Taus/1(tau) -> 1/stiffness/1
  Parallelogram Backlash Compensatior/1(epsilon) -> Mux1/1
  1/stiffness/1 -> comp perc/1  "epsilon"
  comp perc/1 -> Mux1/2, wrist compensation/1(epsilon)
  padding 2 for wrist and gripper/1 -> Mux1/4
  wrist compensation/1(q_wrist) -> Mux1/3
  Multiport Switch/1 -> epsilon/1
  Mux1/1 -> Multiport Switch/2
  compensation mode/1 -> Multiport Switch/1, [comp_mode]
  RR Act Compensation/1(eps) -> Multiport Switch/3
  q_eps_ref/1 -> q_eps 5th order poly/1(q_eps_ref)
  Compare To Constant/1 -> q_eps 5th order poly/2(enable)
  q_eps 5th order poly/1(q_eps_des) -> Multiport Switch/4
  [comp_mode] -> Compare To Constant/1
  psi dot/1 -> get q_dot sign/1(conf_space_dot)
  get q_dot sign/1(q_dot) -> q_dot_sign/1, RR Act Compensation/2(q_dot)
  q_dot_sign/1 -> q dot sgn/1

== system irep_force_control_simu_v2/Trajectory Planner/Right Arm/High Level/Configuration Space ==
  Enable : EnablePort
  Enable Parallelogram : Constant  Value=0  SampleTime=dt
  Enable Stem : Constant  Value=0  SampleTime=dt
  Mux : Mux  Inputs=3
  Parallelogram : Subsystem  TreatAsAtomicUnit=on
  Stem : Subsystem  TreatAsAtomicUnit=on
  XYZ : Constant  Value=0  SampleTime=dt
  "b1 dot, psi dot" : Outport  PortDimensions=8  InitialOutput=zeros(8,1)
  wires:
  Mux/1 -> "b1 dot, psi dot"/1
  Enable Parallelogram/1 -> Parallelogram/Enable
  Enable Stem/1 -> Stem/Enable
  Stem/1(psi dot) -> Mux/3
  Parallelogram/1(b1) -> Mux/2
  XYZ/1 -> Mux/1

== system irep_force_control_simu_v2/Trajectory Planner/Right Arm/High Level/Inverse Istantaneous Kinematics ==
  PSI dot : Inport
  sensors : Inport  Port=2
  Master : Inport  Port=3
  5-Bar Inverse Kinematics : MATLAB Function  TreatAsAtomicUnit=on
  Bus Creator : BusCreator  Inputs=3
  Bus Selector : BusSelector  OutputSignals=q.Parker insertion stage
  Coordination Module : Subsystem
  Demux : Demux  Outputs=[1 2 5]
  Enable Gripper : Constant  Value=0  SampleTime=dt
  Integrator 3 : DiscreteIntegrator  InitialCondition=[x0_parallelogram z0_parallelogram]  SampleTime=dt  LimitOutput=on  UpperSaturationLimit=[x0_parallelogram_max z0_parallelogram_max]  LowerSaturationLimit=[x0_parallelogram z0_parallelogram]
  Integrator 4 : DiscreteIntegrator  InitialCondition=[pi/2;0;pi/2;0;0]  SampleTime=dt  LimitOutput=on  UpperSaturationLimit=[theta_max inf theta_max inf wrist_max]  LowerSaturationLimit=[theta_min1 -inf theta_min2 -inf wrist_min]
  Jaw Open/Close Module : Subsystem  TreatAsAtomicUnit=on
  Mux : Mux
  Saturation : Saturate  UpperLimit=30  LowerLimit=0
  Snake inverse position : MATLAB Function  TreatAsAtomicUnit=on
  q des : Outport
  conf space : Outport  Port=2  PortDimensions=8
  b0_dot_right : Outport  Port=3
  wires:
  5-Bar Inverse Kinematics/1(q) -> Coordination Module/2(q par)
  Integrator 3/1 -> [b1], 5-Bar Inverse Kinematics/1(b1), Coordination Module/1(b1)  "b1 curr"
  Coordination Module/1(q1) -> Saturation/1  "q1"
  Jaw Open/Close Module/1(q9) -> Mux/4  "q9"
  Mux/1 -> q des/1
  PSI dot/1 -> Demux/1
  Bus Creator/1 -> conf space/1
  Integrator 4/1 -> Bus Creator/3, Snake inverse position/1(psi)  "psi curr"
  Coordination Module/2("q2, q3") -> Mux/2  "q2, q3"
  sensors/1 -> Bus Selector/1
  Enable Gripper/1 -> Jaw Open/Close Module/Enable
  [b1] -> Bus Creator/2
  Bus Selector/1 -> Bus Creator/1  "<Parker insertion stage>"
  Demux/3 -> Integrator 4/1  "psi dot"
  Demux/2 -> Integrator 3/1  "b1 dot"
  Demux/1 -> b0_dot_right/1  "b0 dot"
  Saturation/1 -> Mux/1
  Snake inverse position/1(q) -> Mux/3
  Master/1 -> Jaw Open/Close Module/1(sensors)

== system irep_force_control_simu_v2/Trajectory Planner/Right Arm/High Level/Task Space ==
  note: IREP Task Space Module v 0.2 - © 2011 Andrea Bajo, Nabil Simaan
  Master : Inport
  "b1 curr, psi curr" : Inport  Port=2
  sensors : Inport  Port=3
  Enable : EnablePort
  Bus Creator : BusCreator  Inputs=2
  Bus Selector : BusSelector  OutputSignals=p in world,R in world
  Compute Weigths : Subsystem  TreatAsAtomicUnit=on
  Desired Twist Module : Subsystem
  Direct Kinematics IREP : Subsystem  TreatAsAtomicUnit=on
  Jxpsi Inverse IREP : Subsystem  TreatAsAtomicUnit=on
  Receive Desired Pose from MTM : Subsystem
  pose cur quat : MATLAB Function  TreatAsAtomicUnit=on
  right task space scope : Subsystem
  "b0 dot, b1 dot, psi dot" : Outport  PortDimensions=8  InitialOutput=zeros(8,1)
  current_pose : Outport  Port=2  PortDimensions=7  InitialOutput=[zeros(3,1);1;0;0;0]
  wires:
  "b1 curr, psi curr"/1 -> Direct Kinematics IREP/1("b1, psi"), Compute Weigths/2(conf space), Jxpsi Inverse IREP/3("b1, psi")
  Receive Desired Pose from MTM/1("pose, flags") -> Desired Twist Module/2(des pose), [R_Pose_des]
  Direct Kinematics IREP/1(Current Pose) -> Desired Twist Module/1(current pose), Bus Selector/1
  Master/1 -> Receive Desired Pose from MTM/1(Master)
  Jxpsi Inverse IREP/1(conf dot des) -> "b0 dot, b1 dot, psi dot"/1
  Desired Twist Module/1(x des) -> Jxpsi Inverse IREP/1(x des)
  Compute Weigths/1(weights) -> Jxpsi Inverse IREP/2(weights)
  [R_Pose_des] -> right task space scope/1(des)
  sensors/1 -> Compute Weigths/1(sensors)
  Bus Creator/1 -> current_pose/1
  Bus Selector/1 -> Bus Creator/1  "<p in world>"
  Bus Selector/2 -> pose cur quat/1(R)  "<R in world>"
  pose cur quat/1(quat) -> Bus Creator/2

== system irep_force_control_simu_v2/Trajectory Planner/Right Arm/High Level/delay ==
  In1 : Inport
  Bus Creator : BusCreator
  Demux : Demux  Outputs=[1,2,5,1]
  Unit Delay : UnitDelay  InitialCondition=zeros(9,1)  SampleTime=-1
  Out1 : Outport
  wires:
  Unit Delay/1 -> Demux/1
  In1/1 -> Unit Delay/1
  Bus Creator/1 -> Out1/1
  Demux/1 -> Bus Creator/1  "q1"
  Demux/2 -> Bus Creator/2  "q2;q3"
  Demux/3 -> Bus Creator/3  "q_snake"
  Demux/4 -> Bus Creator/4  "q9"

== system irep_force_control_simu_v2/Trajectory Planner/Right Arm/Low Level/Home Procedure ==
  sensors : Inport
  Enable : EnablePort
  Bus Selector : BusSelector  OutputSignals=A/D signals.right arm pots
  Demux : Demux  Outputs=[9 1]
  Fine Homing - Integral Control : Subsystem
  Fine_Rough_Homing_Switch : MATLAB Function  TreatAsAtomicUnit=on
  Homing Completion : MATLAB Function  TreatAsAtomicUnit=on
  Homing Direction : Gain  Gain=diag(RightArmHomingDirectionVector)  Multiplication=Matrix(K*u)  SampleTime=dt
  HomingFineEps : Constant  Value=HomingFineEps  SampleTime=dt
  HomingRoughEps : Constant  Value=HomingRoughEps  SampleTime=dt
  HomingRoughVelocity : Constant  Value=HomingRoughVelocity  SampleTime=dt
  Select Homing Joint : Gain  Gain=diag([1;1;1;1;1;1;1;0;0])  Multiplication=Matrix(K*u)  SampleTime=dt
  Sum : Sum  Inputs=|+-  SampleTime=dt
  Sum1 : Sum  Inputs=|++
  Terminator : Terminator
  Terminator1 : Terminator
  Unit Delay : UnitDelay  InitialCondition=zeros(9,1)  SampleTime=-1
  Unit Delay1 : UnitDelay  InitialCondition=false(9,1)  SampleTime=-1
  dt : Constant  Value=dt  SampleTime=dt
  home voltage : Constant  Value=right_arm_home_voltage  SampleTime=dt
  q des : Outport  InitialOutput=zeros(9,1)
  wires:
  sensors/1 -> Bus Selector/1
  Sum/1 -> Select Homing Joint/1
  home voltage/1 -> Sum/1
  Bus Selector/1 -> Demux/1  "<right arm pots>"
  Demux/1 -> Sum/2
  Demux/2 -> Terminator/1
  Homing Completion/1(Homed) -> Terminator1/1
  Select Homing Joint/1 -> Homing Direction/1
  HomingRoughVelocity/1 -> Fine_Rough_Homing_Switch/4(HomingVel)
  Unit Delay1/1 -> Fine_Rough_Homing_Switch/6(PrevHomedJoint)
  Fine_Rough_Homing_Switch/3(HomedJoint) -> Unit Delay1/1
  HomingRoughEps/1 -> Fine_Rough_Homing_Switch/3(ERROR_eps)
  dt/1 -> Fine_Rough_Homing_Switch/2(dt)
  Unit Delay/1 -> Fine_Rough_Homing_Switch/5(q_cur)
  Fine_Rough_Homing_Switch/2(q_des) -> Unit Delay/1, Sum1/2
  Fine_Rough_Homing_Switch/1(EnableFineHoming) -> Fine Homing - Integral Control/Enable
  Fine Homing - Integral Control/1(q_des_fine) -> Sum1/1
  Sum1/1 -> q des/1
  Homing Direction/1 -> Homing Completion/1(u), Fine_Rough_Homing_Switch/1(error), Fine Homing - Integral Control/1(error)
  HomingFineEps/1 -> Homing Completion/2(EPS)

== system irep_force_control_simu_v2/Trajectory Planner/Right Arm/Low Level/Joint Space ==
  Enable : EnablePort
  q desired : Constant  Value=zeros(9,1)  SampleTime=dt
  q des : Outport
  wires:
  q desired/1 -> q des/1

== system irep_force_control_simu_v2/Trajectory Planner/UDP_SendTo_MTM/Left_UDP/pose convert ==
  pose_q : Inport
  Bus Creator : BusCreator  Inputs=2
  Bus Selector4 : BusSelector  OutputSignals=p in world,quat
  Quaternion To Rotation : MATLAB Function  TreatAsAtomicUnit=on
  pose_R : Outport
  wires:
  Bus Creator/1 -> pose_R/1
  Bus Selector4/1 -> Bus Creator/1  "<p in world>"
  Quaternion To Rotation/1(R) -> Bus Creator/2  "R in world"
  pose_q/1 -> Bus Selector4/1
  Bus Selector4/2 -> Quaternion To Rotation/1(quat)  "<quat>"
